simulink model "ps8"  (R2020b)
settings: Solver=VariableStepAuto  StartTime=0.0  StopTime=10.0  RelTol=1e-3
libraries: pid_lib x1
settings Model: Creator=prana  LastModifiedBy=prana

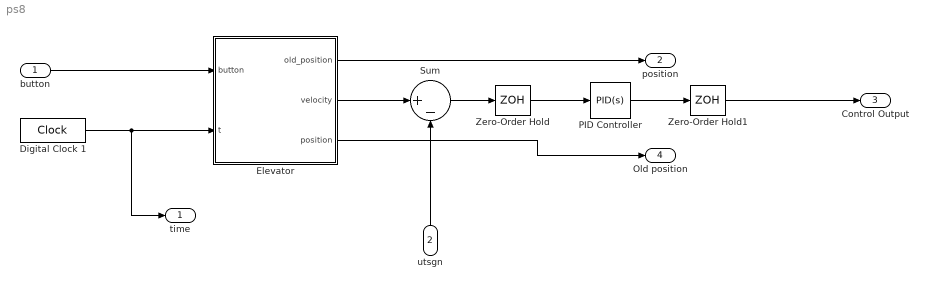
== system ps8 ==
  button : Inport
  utsgn : Inport  Port=2
  Digital Clock 1 : DigitalClock  SampleTime=10
  "Elevator " : Stateflow chart  TreatAsAtomicUnit=on
  PID Controller : pid_lib/PID Controller  Controller=PID  Form=Parallel  TimeDomain=Continuous-time  UseExternalTs=off  SampleTime=-1  IntegratorMethod=Forward Euler  FilterMethod=Forward Euler  ControllerParametersSource=internal  P=1  I=1  D=0  UseFilter=on  N=100  TunerSelectOption=Transfer Function Based (PID Tuner App)  InitialConditionSource=internal  InitialConditionForIntegrator=0  InitialConditionForFilter=0  DifferentiatorICPrevScaledInput=0  ExternalReset=none  TrackingMode=off  Kt=1  LimitOutput=off  SatLimitsSource=internal  UpperSaturationLimit=inf  LowerSaturationLimit=-inf  LinearizeAsGain=on  AntiWindupMode=none  Kb=1  POutMin=[]  POutMax=[]  IOutMin=[]  IOutMax=[]  DOutMin=[]  DOutMax=[]  NOutMin=[]  NOutMax=[]  SumOutMin=[]  SumOutMax=[]  SaturationOutMin=[]  SaturationOutMax=[]  PParamMin=[]  PParamMax=[]  IParamMin=[]  IParamMax=[]  DParamMin=[]  DParamMax=[]  NParamMin=[]  NParamMax=[]  KbParamMin=[]  KbParamMax=[]  KtParamMin=[]  KtParamMax=[]  KbOutMin=[]  KbOutMax=[]  KtOutMin=[]  KtOutMax=[]  IntegratorOutMin=[]  IntegratorOutMax=[]  FilterOutMin=[]  FilterOutMax=[]  SumI1OutMin=[]  SumI1OutMax=[]  SumI2OutMin=[]  SumI2OutMax=[]  SumI3OutMin=[]  SumI3OutMax=[]  SumI4OutMin=[]  SumI4OutMax=[]  SumDOutMin=[]  SumDOutMax=[]  DifferentiatorOutMin=[]  DifferentiatorOutMax=[]  FilterDiffOutCoefMin=[]  FilterDiffOutCoefMax=[]  ReciprocalOutMin=[]  ReciprocalOutMax=[]  SumDenOutMin=[]  SumDenOutMax=[]  SumNumOutMin=[]  SumNumOutMax=[]  DivideOutMin=[]  DivideOutMax=[]  UdiffTsProdOutMin=[]  UdiffTsProdOutMax=[]  NTsProdOutMin=[]  NTsProdOutMax=[]  UintegralTsProdOutMin=[]  UintegralTsProdOutMax=[]  UngainTsProdOutMin=[]  UngainTsProdOutMax=[]  IntegratorContinuousStateAttributes=''  IntegratorStateMustResolveToSignalObject=off  IntegratorRTWStateStorageClass=Auto  FilterContinuousStateAttributes=''  FilterStateMustResolveToSignalObject=off  FilterRTWStateStorageClass=Auto  ParallelPVariant=InternalParameters  IdealPVariant=Disabled  IVariant=InternalParameters  DVariant=InternalParameters  IntegratorVariant=Continuous  SatVariant=Disabled  AWVariant=Passthrough  PCopyVariant=Disabled  TRVariant=Disabled  FdbkBlocksVariant=Forward  IdealPFdbkVariant=Disabled  SatFdbkVariant=Disabled  DerivativeFilterVariant=ContFilter  NVariant=InternalParameters  NCopyVariant=Disabled  FilterICVariant=InternalICsFilter  IntegratorICVariant=InternalICs  ExternalResetVariant=Disabled  TRSumVariant=Passthrough  SumFdbkVariant=Disabled  SumVariant=Sum_PID  TsampFilterVariant=InternalTs  TsampNgainVariant=Passthrough  TsampIntegralVariant=Passthrough  ExternalSaturationOutDataTypeStr=Inherit: Same as second input
  Sum : Sum  Inputs=|+-
  Zero-Order Hold : ZeroOrderHold  SampleTime=-1
  Zero-Order Hold1 : ZeroOrderHold  SampleTime=-1
  time : Outport
  position : Outport  Port=2
  Control Output : Outport  Port=3
  Old position : Outport  Port=4
  wires:
  Digital Clock 1/1 -> time/1, "Elevator "/2(t)
  button/1 -> "Elevator "/1(button)
  "Elevator "/2(velocity) -> Sum/1
  utsgn/1 -> Sum/2
  "Elevator "/1(old_position) -> position/1
  "Elevator "/3(position) -> Old position/1
  Sum/1 -> Zero-Order Hold/1
  Zero-Order Hold/1 -> PID Controller/1
  Zero-Order Hold1/1 -> Control Output/1
  PID Controller/1 -> Zero-Order Hold1/1

== stateflow chart ps8/Elevator  ==
  state Elevator
    note: % runs elevator motor if a button has been pushed
    note: % if on the top floor, and button is less than zero,
        | % or if on ground floor, and button is more than zero,
        | % run elevator
    state ReadKeyboard
    state RunMotor
      en:
      position=(velocity*t) +old_position
      ex:
      old_position = position;
      velocity = button;
    state ReadKeyboard2
    note: % if on the top floor, and button is more than zero,
        | % or if on ground floor, and button is less than zero,
        | % stop elevator
    state Stop
      en:
      velocity=0;
    state Hold
    ReadKeyboard -> RunMotor [order 2] : [(button>0&&position<100)||(button<0&&position>0)]
    RunMotor -> ReadKeyboard [order 1] : [(button>0&&position<1000)||(button<0&&position>0)]
    Hold -> ReadKeyboard [order 2] : [button>0&&position<500]
    ReadKeyboard -> Hold [order 1] : [(button>0&&position>1000)||(button<0&&position<0)]
    ReadKeyboard2 -> RunMotor
    RunMotor -> ReadKeyboard2 [order 3]
    RunMotor -> Stop [order 2] : [position>1000||position<0]
    Hold -> ReadKeyboard2 [order 1] : [button<0&&position>0]
    Stop -> Hold
    Hold -> Stop [order 3]
    (default) -> Hold
  data: button input size=1; old_position output size=1; velocity output size=1; position output size=1; t input size=1
